simulink model "vehicle"  (R2018b)
settings: Solver=VariableStepAuto  StartTime=0.0  StopTime=10.0  RelTol=1e-3
values from neighbouring files (symbols this model uses):
  g = 9.81    [dane.m]    (also in untitled.m)
  m_v = 1200    [dane.m]
  r_w = 0.3    [dane.m]    (also in untitled.m)
  v0 = 28    [dane.m]
settings Model: Creator=lpa1  LastModifiedBy=lpa1

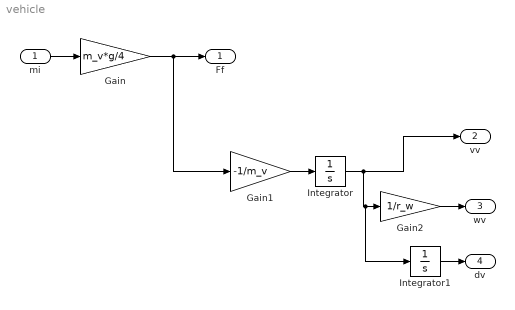
== system vehicle ==
  mi : Inport
  Gain : Gain  Gain=m_v*g/4
  Gain1 : Gain  Gain=-1/m_v
  Gain2 : Gain  Gain=1/r_w
  Integrator : Integrator  InitialCondition=v0  LimitOutput=on  UpperSaturationLimit=1000  LowerSaturationLimit=0.001
  Integrator1 : Integrator
  "Ff " : Outport
  vv : Outport  Port=2
  wv : Outport  Port=3
  "dv " : Outport  Port=4
  wires:
  mi/1 -> Gain/1
  Gain/1 -> Gain1/1, "Ff "/1
  Gain1/1 -> Integrator/1
  Integrator/1 -> Integrator1/1, Gain2/1, vv/1
  Gain2/1 -> wv/1
  Integrator1/1 -> "dv "/1
